simulink model "NonlinearDynamic"  (R2020b)
settings: Solver=VariableStepAuto  StartTime=0.0  StopTime=10.0  RelTol=1e-3
values from neighbouring files (symbols this model uses):
  bw = 0.01    [VehicleModelDictionary.sldd]    (also in VehicleParameters.m; VehicleParametersDictionary.sldd)
  g = 9.80665    [VehicleModelDictionary.sldd]    (also in VehicleParameters.m; VehicleParametersDictionary.sldd)
  Ib = 0.00290817    [VehicleModelDictionary.sldd]    (also in VehicleParameters.m; VehicleParametersDictionary.sldd)
  Iw = 2.78742E-5    [VehicleModelDictionary.sldd]    (also in VehicleParameters.m = 2.78742e-05; VehicleParametersDictionary.sldd)
  l = 0.06    [VehicleModelDictionary.sldd]    (also in VehicleParameters.m; VehicleParametersDictionary.sldd)
  mb = 0.5    [VehicleModelDictionary.sldd]    (also in VehicleParameters.m; VehicleParametersDictionary.sldd)
  mw = 0.064    [VehicleModelDictionary.sldd]    (also in VehicleParameters.m; VehicleParametersDictionary.sldd)
  rw = 0.032    [VehicleModelDictionary.sldd]    (also in VehicleParameters.m; VehicleParametersDictionary.sldd)
undefined symbols (not defined in the file or in its folder): x0
settings Model: DataDictionary=VehicleParametersDictionary.sldd  Creator=Gonzalo Fernández  LastModifiedBy=Gonzalo Fernández

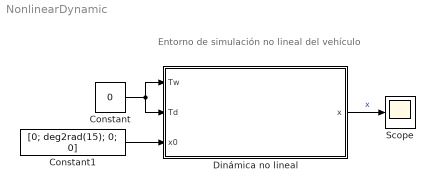
== system NonlinearDynamic ==
  note: Entorno de simulación no lineal del vehículo
  Constant : Constant  Value=0
  Constant1 : Constant  Value=[0; deg2rad(15); 0; 0]
  Dinámica no lineal : Subsystem
  Scope : Scope
  wires:
  Constant/1 -> Dinámica no lineal/2(Td), Dinámica no lineal/1(Tw)
  Dinámica no lineal/1(x) -> Scope/1  "x"
  Constant1/1 -> Dinámica no lineal/3(x0)

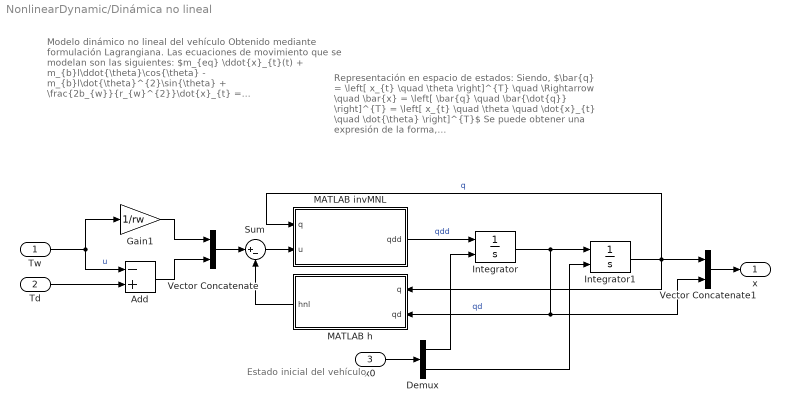
== system NonlinearDynamic/Dinámica no lineal ==
  note: Estado inicial del vehículo
  note: Representación en espacio de estados:
      | Siendo,
      | $\bar{q} = \left[ x_{t} \quad \theta \right]^{T} \quad \Rightarrow \quad \bar{x} = \left[ \bar{q} \quad \bar{\dot{q}} \right]^{T} = \left[ x_{t} \quad \theta \quad \dot{x}_{t} \quad \dot{\theta} \right]^{T}$
      | Se puede obtener una expresión de la forma,
      |
      | $^{NL}\mathbb{E}(\bar{q})\cdot \bar{\ddot{q}} + h(\bar{q}, \bar{\dot{q}}) = \mathbb{H}_{T} \cdot \bar{u}$
  note: Modelo dinámico no lineal del vehículo
      |
      | Obtenido mediante formulación Lagrangiana.
      | Las ecuaciones de movimiento que se modelan son las siguientes:
      | $m_{eq} \ddot{x}_{t}(t) + m_{b}l\ddot{\theta}\cos{\theta} - m_{b}l\dot{\theta}^{2}\sin{\theta} + \frac{2b_{w}}{r_{w}^{2}}\dot{x}_{t} = \frac{1}{r_{w}}T_{w}\\ m_{b}l\ddot{x}_{t}\cos{\theta} + I_{eq}\ddot{\theta} - m_{b}gl\sin{\theta} = -T_{w} + T_{d}$
      | Donde,
      | $m_{eq} = m_{b} + 2m_{w} + \frac{2I_{w}}{r_{w}^{2}} \quad\quad I_{eq} = I_{b} + m_{b}l^{2}$
  Tw : Inport
  Td : Inport  Port=2
  x0 : Inport  Port=3  PortDimensions=[4, 1]
  Add : Sum  Inputs=-+
  Demux : Demux  Outputs=2
  Gain1 : Gain  Gain=1/rw
  Integrator : Integrator  InitialConditionSource=external  InitialCondition=x0(3:4)
  Integrator1 : Integrator  InitialConditionSource=external  InitialCondition=x0(1:2)
  MATLAB h : MATLAB Function  TreatAsAtomicUnit=on
  MATLAB invMNL : MATLAB Function  TreatAsAtomicUnit=on
  Sum : Sum  Inputs=|+-
  Vector Concatenate : Concatenate
  Vector Concatenate1 : Concatenate
  x : Outport
  wires:
  Sum/1 -> MATLAB invMNL/2(u)
  Vector Concatenate/1 -> Sum/1
  MATLAB invMNL/1(qdd) -> Integrator/1  "qdd"
  MATLAB h/1(hnl) -> Sum/2
  Gain1/1 -> Vector Concatenate/1
  Tw/1 -> Add/1, Gain1/1  "u"
  Add/1 -> Vector Concatenate/2
  Integrator/1 -> Integrator1/1, Vector Concatenate1/2, MATLAB h/2(qd)  "qd"
  Integrator1/1 -> Vector Concatenate1/1, MATLAB h/1(q), MATLAB invMNL/1(q)  "q"
  Vector Concatenate1/1 -> x/1
  Td/1 -> Add/2
  x0/1 -> Demux/1
  Demux/1 -> Integrator/2
  Demux/2 -> Integrator1/2

== matlab function NonlinearDynamic/Dinámica no lineal/MATLAB invMNL ==
  data: q input; u input; qdd output; mw parameter; Iw parameter; rw parameter; mb parameter; l parameter; Ib parameter
function qdd = invENL(q, u, mw, Iw, rw, mb, l, Ib)
ENL = [
    2*mw + 2*Iw/rw^2 + mb,  mb*l*cos(q(2));
    mb*l*cos(q(2)),         Ib + mb*l^2
];
qdd = ENL\u; % inv(MNL)*u

== matlab function NonlinearDynamic/Dinámica no lineal/MATLAB h ==
  data: q input; hnl output; qd input; bw parameter; rw parameter; mb parameter; l parameter; g parameter
function hnl = h(q, qd, bw, rw, mb, l, g)
hnl = [
    2*bw/rw^2*qd(1) - mb*l*qd(2)^2*sin(q(2));
    -mb*g*l*sin(q(2))
];
